simulink model "Simple_MIMO_Trying"  (R2018b)
settings: Solver=VariableStepAuto  StartTime=0.0  StopTime=10.0  RelTol=1e-3
undefined symbols (not defined in the file): doppler, j
libraries: commdigbbndpm3 x2, commrandsrc3 x2, commsink2 x2, commmimo x2, commlibv2 x1, commchan3 x1, commeq2 x1, commsource2 x1
settings Model: Creator=nhj94  LastModifiedBy=nhj94

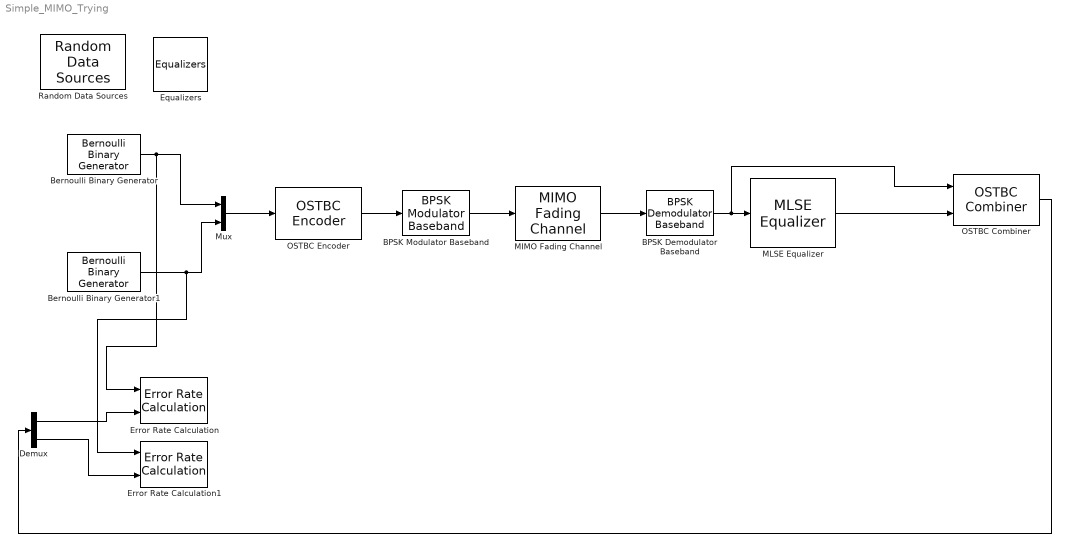
== system Simple_MIMO_Trying ==
  BPSK Demodulator Baseband : commdigbbndpm3/BPSK Demodulator Baseband  DecType=Hard decision  VarSource=Dialog  Variance=1  Ph=0  outDtype=Inherit via internal rule  derotateFactorWordLen=16  derotateFactorDataTypeStr=Inherit: Same word length as input  derotateFactorLastDataTypeStr=Inherit: Same word length as input
  BPSK Modulator Baseband : commdigbbndpm3/BPSK Modulator Baseband  Ph=0  outDtype=double  outWordLen=16  outUDDataType=sfix(16)  outFracLenMode=Best precision  outFracLen=15  outDataTypeStr=double  outLastDataTypeStr=double
  Bernoulli Binary Generator : commrandsrc3/Bernoulli Binary Generator  ProbabilityOfZero=0.5  SeedSource=Auto  Seed=0  SampleTime=1  SamplesPerFrame=100  OutputDataType=double  SimulateUsing=Interpreted execution
  Bernoulli Binary Generator1 : commrandsrc3/Bernoulli Binary Generator  ProbabilityOfZero=0.5  SeedSource=Auto  Seed=0  SampleTime=1  SamplesPerFrame=100  OutputDataType=double  SimulateUsing=Interpreted execution
  Demux : Demux  Outputs=2
  Equalizers : commlibv2/Equalizers
      settings: SourceProductName=Communications System Toolbox  SourceProductBaseCode=CM
  Error Rate Calculation : commsink2/Error Rate Calculation  N=0  st_delay=0  cp_mode=Entire frame  subframe=[]  PMode=Workspace  WsName=ErrorVec  RsMode2=off  stop=off  numErr=100  maxBits=1e6
  Error Rate Calculation1 : commsink2/Error Rate Calculation  N=0  st_delay=0  cp_mode=Entire frame  subframe=[]  PMode=Workspace  WsName=ErrorVec  RsMode2=off  stop=off  numErr=100  maxBits=1e6
  MIMO Fading Channel : commchan3/MIMO Fading Channel  InheritSampleRate=on  SampleRate=1  PathDelays=0  AveragePathGains=0  NormalizePathGains=on  FadingDistribution=Rayleigh  KFactor=3  DirectPathDopplerShift=0  DirectPathInitialPhase=0  MaximumDopplerShift=0.001  DopplerSpectrum=doppler('Jakes')  SpatialCorrelationSpecification=None  SpatialCorrelationMatrix=[1 0 0 0; 0 1 0 0; 0 0 1 0; 0 0 0 1]  NumTransmitAntennas=2  NumReceiveAntennas=2  TransmitCorrelationMatrix=[1 0; 0 1]  ReceiveCorrelationMatrix=[1 0; 0 1]  AntennaSelection=Off  NormalizeChannelOutputs=on  SimulateUsing=Interpreted execution  FadingTechnique=Filtered Gaussian noise  NumSinusoids=48  InitialTimeSource=Property  InitialTime=0  ChannelInterpolationMethod=Polyphase  RandomStream=mt19937ar with seed  Seed=73  PathGainsOutputPort=off  Visualization=Off  AntennaPairsToDisplay=[ 1, 1 ]  PathsForDopplerDisplay=1  SamplesToDisplay=25%
      settings: SourceProductName=Communications System Toolbox  SourceProductBaseCode=CM
  MLSE Equalizer : commeq2/MLSE Equalizer  specchan=Dialog  chancoeff=[1 0.7 0.5 0.3]'  constpts=[1+j -1+j -1-j 1-j]  tbdepth=21  opmode=Reset every frame  enpreamble=off  preamble=[0 3 2 1]  enpostamble=off  postamble=[0 2 3 1]  numsamp=1  reset=off
      settings: SourceProductName=Communications System Toolbox  SourceProductBaseCode=CM
  Mux : Mux  Inputs=2
  OSTBC Combiner : commmimo/OSTBC Combiner  numTx=2  rate=3/4  numRx=1  roundingMode=Floor  overflowMode=Wrap  OvFlMode=off  OvFlModeLastStrValue=off  crossProductWordLen=32  crossProductFracLen=16  crossSumWordLen=32  crossSumFracLen=16  egyProductWordLen=32  egyProductFracLen=16  egySumWordLen=32  egySumFracLen=16  divisionWordLen=32  divisionFracLen=16  divisionDataTypeStr=Inherit: Same as accumulator  divisionLastDataTypeStr=Inherit: Same as accumulator
      settings: SourceProductName=Communications System Toolbox  SourceProductBaseCode=CM
  OSTBC Encoder : commmimo/OSTBC Encoder  numTx=2  rate=3/4  overflowMode=Wrap  OvFlMode=off  OvFlModeLastStrValue=off
      settings: SourceProductName=Communications System Toolbox  SourceProductBaseCode=CM
  Random Data Sources : commsource2/Random Data Sources
      settings: SourceProductName=Communications System Toolbox  SourceProductBaseCode=CM
  wires:
  Bernoulli Binary Generator/1 -> Error Rate Calculation/1, Mux/1
  Bernoulli Binary Generator1/1 -> Error Rate Calculation1/1, Mux/2
  Mux/1 -> OSTBC Encoder/1
  OSTBC Encoder/1 -> BPSK Modulator Baseband/1
  BPSK Modulator Baseband/1 -> MIMO Fading Channel/1
  MIMO Fading Channel/1 -> BPSK Demodulator Baseband/1
  BPSK Demodulator Baseband/1 -> OSTBC Combiner/1, MLSE Equalizer/1
  MLSE Equalizer/1 -> OSTBC Combiner/2
  OSTBC Combiner/1 -> Demux/1
  Demux/1 -> Error Rate Calculation/2
  Demux/2 -> Error Rate Calculation1/2
